simulink model "PPMSFartoystyring"  (R2017b)
settings: Solver=ode45  StartTime=tstart  StopTime=tstop  RelTol=1e-3  EnableMultiTasking=on
values from neighbouring files (symbols this model uses):
  c = 1    [task27.m]
  p0 = [1000, 700]    [task27.m]
  psi0 = deg2rad(60)    [task27.m]
  r0 = 0    [task27.m]
  tsamp = 10    [task27.m]
  v0 = [6.63 0]'    [task27.m]
undefined symbols (not defined in the file or in its folder): chi2psi, delta_max, heading_controller, K_iu, K_psi, K_pu, L_pp, msfartoystyring, n_max, speed_controller, T_psi, track_dist, U2u, U_t, WP
settings Model: ExtModeAutoUpdateStatusClock=off  Creator=christh  LastModifiedBy=sigtot
settings DataIOCC: LimitDataPoints=on  SaveFormat=Array
settings OptimizationCC: ExpressionDepthLimit=2147483647  InitFltsAndDblsToZero=on  LifeSpan=inf
settings DebuggingCC: UnderspecifiedInitializationDetection=Classic  MergeDetectMultiDrivingBlocksExec=none  SolverPrmCheckMsg=warning  FcnCallInpInsideContextMsg=warning  StateNameClashWarn=warning  SFUnexpectedBacktrackingDiag=warning  SFNoUnconditionalDefaultTransitionDiag=warning
settings HardwareCC: ProdBitPerPointer=32  ProdBitPerSizeT=32  ProdBitPerPtrDiffT=32  ProdLargestAtomicFloat=None  ProdIntDivRoundTo=Undefined  ProdEndianess=Unspecified  ProdWordSize=32  ProdHWDeviceType=32-bit Generic
settings ModelReferenceCC: PropagateSignalLabelsOutOfModel=off
settings CodeAppCC: StateflowObjectComments=on
settings GRTTargetCC: TargetLangStandard=C89/C90 (ANSI)  GeneratePreprocessorConditionals=Disable all  CombineOutputUpdateFcns=off  GRTInterface=on
settings ConfigComp: CovMetricSettings=dw  CovHtmlReporting=on  CovSaveCumulativeToWorkspaceVar=on  CovSaveSingleToWorkspaceVar=on  CovExternalEMLEnable=off

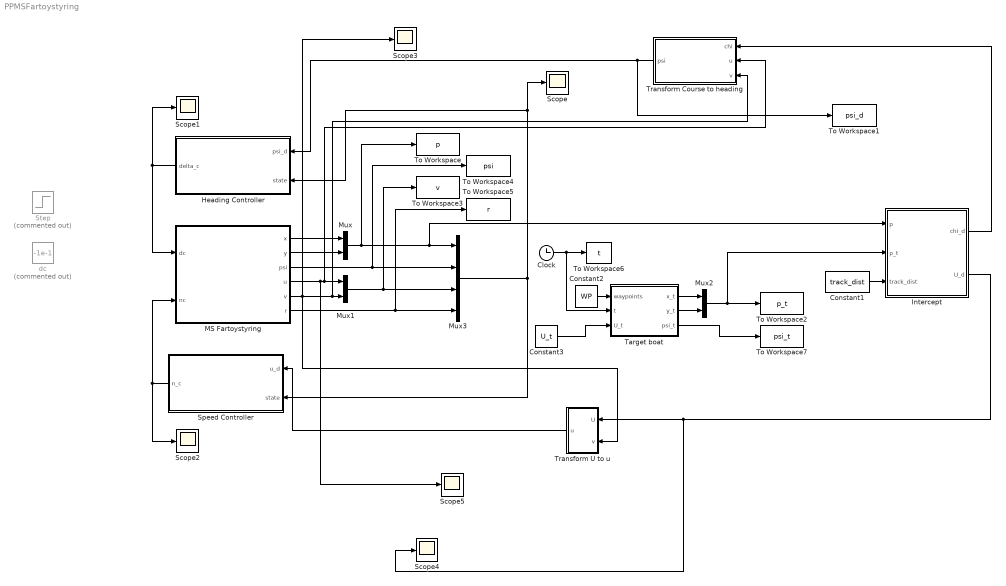
== system PPMSFartoystyring ==
  Clock : Clock
  Constant1 : Constant  Value=track_dist
  Constant2 : Constant  Value=WP
  Constant3 : Constant  Value=U_t
  "Heading Controller " : Subsystem
  Intercept : MATLAB Function  TreatAsAtomicUnit=on
  MS Fartoystyring : Subsystem  mask(MS Fartoystyring for Assignment 3 G&C){x0=p0(1), y0=p0(2), u0=v0(1), v0=v0(2), psi0=psi0, r0=r0, c=c}
      mask prompts: x0 "x(t0) (m)"; y0 "y(t0) (m)"; u0 "u(t0) (m/s)"; v0 "v(t0) (m/s)"; psi0 "psi(t0) (rad)"; r0 "r(t0) (rad/s)"; c "current (0 or 1)"
      mask help:
      | Block corresponding to Figure 1 in the assignment text. Gives the response of the ship.
      |
      | The design speed of MS Fartoystyring is u=8.23 m/s.
      |
      | Input:
      | dc: commanded rudder (rad), dmax=25*pi/180
      | nc: commanded shaft speed (rad/s), nmax=85*2*pi/60
      |
      | Output:
      | x: north pos (m)
      | y: east pos (m)
      | u: surge (m/s)
      | v: sway (m/s)
      | psi: heading (rad)
      | r: yaw (rad/s)
      mask Help: Comments, bugs and help requests can be directed to the TA. Email on course website.
  Mux : Mux  Inputs=2
  Mux1 : Mux  Inputs=2
  Mux2 : Mux  Inputs=2
  Mux3 : Mux
  Scope{,1..5} (6 alike) : Scope
  Speed Controller : Subsystem
  Step : Step  Commented=on  Time=0  After=-deg2rad(25)  SampleTime=0
  Target boat : MATLAB Function  TreatAsAtomicUnit=on
  To Workspace : ToWorkspace  VariableName=p  SampleTime=tsamp
  To Workspace1 : ToWorkspace  VariableName=psi_d  SampleTime=tsamp
  To Workspace2 : ToWorkspace  VariableName=p_t  SampleTime=tsamp
  To Workspace3 : ToWorkspace  VariableName=v  SampleTime=tsamp
  To Workspace4 : ToWorkspace  VariableName=psi  SampleTime=tsamp
  To Workspace5 : ToWorkspace  VariableName=r  SampleTime=tsamp
  To Workspace6 : ToWorkspace  VariableName=t  SampleTime=tsamp
  To Workspace7 : ToWorkspace  VariableName=psi_t  SampleTime=-1
  Transform Course to heading : Subsystem
  Transform U to u : Subsystem
  dc : Constant  Commented=on  Value=-1e-1
  wires:
  Clock/1 -> To Workspace6/1, Target boat/2(t)
  MS Fartoystyring/1(x) -> Mux/1
  MS Fartoystyring/2(y) -> Mux/2
  MS Fartoystyring/4(u) -> Scope5/1, Transform Course to heading/2(u), Mux1/1
  MS Fartoystyring/5(v) -> Transform U to u/2(v), Scope3/1, Transform Course to heading/3(v), Mux1/2
  Mux/1 -> To Workspace/1, Intercept/1(p), Mux3/1
  Mux1/1 -> To Workspace3/1, Mux3/3
  MS Fartoystyring/3(psi) -> To Workspace4/1, Mux3/2
  MS Fartoystyring/6(r) -> To Workspace5/1, Mux3/4
  Mux3/1 -> "Heading Controller "/2(state), Scope/1, Speed Controller/2(state)
  "Heading Controller "/1(delta_c) -> Scope1/1, MS Fartoystyring/1(dc)
  Speed Controller/1(n_c) -> MS Fartoystyring/2(nc), Scope2/1
  Constant2/1 -> Target boat/1(waypoints)
  Transform Course to heading/1(psi) -> "Heading Controller "/1(psi_d), To Workspace1/1
  Transform U to u/1(u) -> Speed Controller/1(u_d)
  Constant3/1 -> Target boat/3(U_t)
  Mux2/1 -> Intercept/2(p_t), To Workspace2/1
  Target boat/1(x_t) -> Mux2/1
  Target boat/2(y_t) -> Mux2/2
  Target boat/3(psi_t) -> To Workspace7/1
  Intercept/1(chi_d) -> Transform Course to heading/1(chi)
  Intercept/2(U_d) -> Scope4/1, Transform U to u/1(U)
  Constant1/1 -> Intercept/3(track_dist)

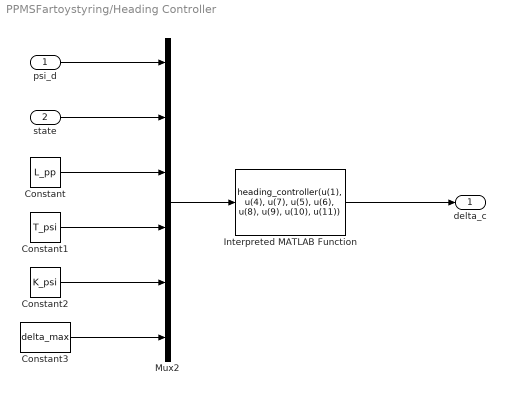
== system PPMSFartoystyring/Heading Controller  ==
  psi_d : Inport
  state : Inport  Port=2
  Constant : Constant  Value=L_pp
  Constant1 : Constant  Value=T_psi
  Constant2 : Constant  Value=K_psi
  Constant3 : Constant  Value=delta_max
  Interpreted MATLAB Function : MATLABFcn  MATLABFcn=heading_controller(u(1), u(4), u(7), u(5), u(6), u(8), u(9), u(10), u(11))
  Mux2 : Mux  Inputs=6
  delta_c : Outport
  wires:
  Constant3/1 -> Mux2/6
  Constant/1 -> Mux2/3
  psi_d/1 -> Mux2/1
  Constant1/1 -> Mux2/4
  state/1 -> Mux2/2
  Interpreted MATLAB Function/1 -> delta_c/1
  Mux2/1 -> Interpreted MATLAB Function/1
  Constant2/1 -> Mux2/5

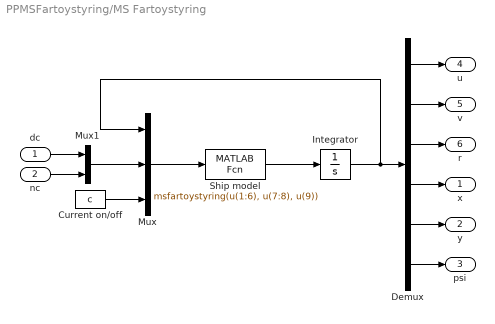
== system PPMSFartoystyring/MS Fartoystyring ==
  dc : Inport
  nc : Inport  Port=2
  Current on/off : Constant  Value=c
  Demux : Demux  Outputs=6
  Integrator : Integrator  InitialCondition=[u0 v0 r0 x0 y0 psi0]'
  Mux : Mux  Inputs=3
  Mux1 : Mux  Inputs=2
  Ship model : MATLABFcn  MATLABFcn=msfartoystyring(u(1:6), u(7:8), u(9))  OutputDimensions=6
  x : Outport
  y : Outport  Port=2
  psi : Outport  Port=3
  u : Outport  Port=4
  v : Outport  Port=5
  r : Outport  Port=6
  wires:
  Integrator/1 -> Mux/1, Demux/1
  Mux1/1 -> Mux/2
  dc/1 -> Mux1/1
  nc/1 -> Mux1/2
  Demux/1 -> u/1
  Demux/2 -> v/1
  Demux/3 -> r/1
  Demux/4 -> x/1
  Demux/5 -> y/1
  Demux/6 -> psi/1
  Current on/off/1 -> Mux/3
  Ship model/1 -> Integrator/1
  Mux/1 -> Ship model/1

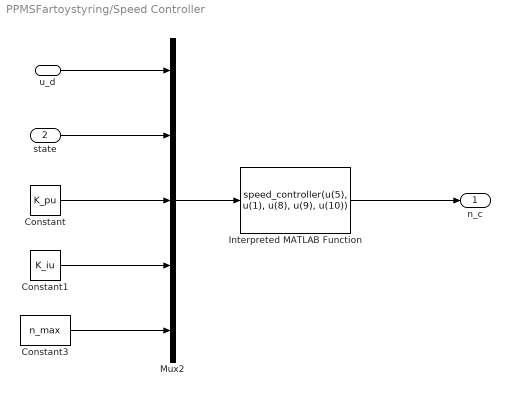
== system PPMSFartoystyring/Speed Controller ==
  u_d : Inport
  state : Inport  Port=2
  Constant : Constant  Value=K_pu
  Constant1 : Constant  Value=K_iu
  Constant3 : Constant  Value=n_max
  Interpreted MATLAB Function : MATLABFcn  MATLABFcn=speed_controller(u(5), u(1), u(8), u(9), u(10))
  Mux2 : Mux  Inputs=5
  n_c : Outport
  wires:
  Interpreted MATLAB Function/1 -> n_c/1
  Mux2/1 -> Interpreted MATLAB Function/1
  u_d/1 -> Mux2/1
  state/1 -> Mux2/2
  Constant/1 -> Mux2/3
  Constant1/1 -> Mux2/4
  Constant3/1 -> Mux2/5

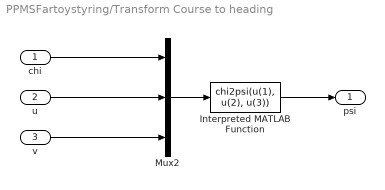
== system PPMSFartoystyring/Transform Course to heading ==
  chi : Inport
  u : Inport  Port=2
  v : Inport  Port=3
  Interpreted MATLAB Function : MATLABFcn  MATLABFcn=chi2psi(u(1), u(2), u(3))
  Mux2 : Mux  Inputs=3
  psi : Outport
  wires:
  u/1 -> Mux2/2
  Mux2/1 -> Interpreted MATLAB Function/1
  v/1 -> Mux2/3
  Interpreted MATLAB Function/1 -> psi/1
  chi/1 -> Mux2/1

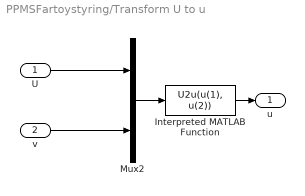
== system PPMSFartoystyring/Transform U to u ==
  U : Inport
  v : Inport  Port=2
  Interpreted MATLAB Function : MATLABFcn  MATLABFcn=U2u(u(1), u(2))
  Mux2 : Mux  Inputs=2
  u : Outport
  wires:
  Mux2/1 -> Interpreted MATLAB Function/1
  U/1 -> Mux2/1
  Interpreted MATLAB Function/1 -> u/1
  v/1 -> Mux2/2

== matlab function PPMSFartoystyring/Target boat ==
  data: waypoints input; x_t output; t input; U_t input; y_t output; psi_t output
function [x_t, y_t, psi_t] = fcn(waypoints, t, U_t)
    chi_t = atan2(waypoints(1, 2) - waypoints(1, 1), waypoints(2, 2) - waypoints(2, 1));
    psi_t = chi_t; % Zero crab angle for target
    x_t = waypoints(1, 2) + sin(chi_t) * U_t * t;
    y_t = waypoints(2, 2) + cos(chi_t) * U_t * t;
end

== matlab function PPMSFartoystyring/Intercept ==
  data: chi_d output; p input; U_d output; p_t input; track_dist input
function [chi_d, U_d] = intercept(p, p_t, track_dist)
delta_x = p_t(1) - p(1); 
delta_y = p_t(2) - p(2); 

chi_d = atan2(delta_y, delta_x); 
U_d = 7;
if (p(1) - p_t(1))^2 + (p(2) - p_t(2))^2 < track_dist^2
    U_d = 2;
end
